simulink library "Driver_Drive_Cycle"  (R2026a)
settings: Solver=VariableStepAuto
undefined symbols (not defined in the file): Driver, Maneuver
Description:
  | Component of Simscape Vehicle Templates Library
  | 
  | Copyright 2018-2026 The MathWorks, Inc.
settings Model: Creator=smiller  LastModifiedBy=smiller

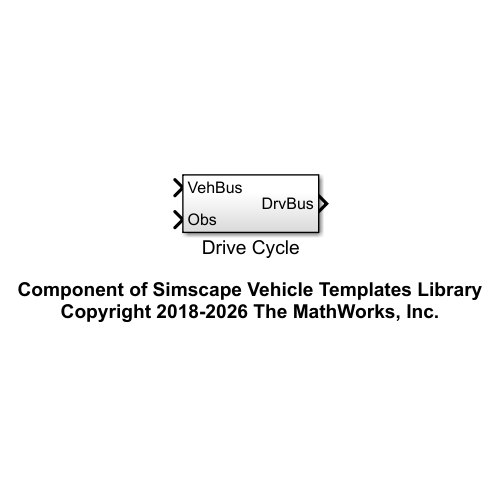
[thumbnail: Simulink's stored preview of the top-level diagram]
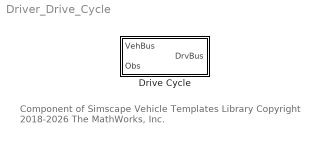
== system Driver_Drive_Cycle ==
  note: Component of Simscape Vehicle Templates Library
      | Copyright 2018-2026 The MathWorks, Inc.
  Drive Cycle : Subsystem  VariantControl=Drive_Cycle

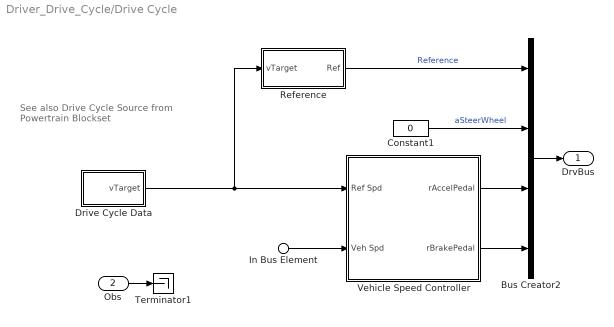
== system Driver_Drive_Cycle/Drive Cycle ==
  note: See also Drive Cycle Source
      | from Powertrain Blockset
  In Bus Element : Inport  PortName=VehBus  Element=Chassis.Body.CG.vx
  Obs : Inport  Port=2
  Bus Creator2 : BusCreator  Inputs=4
  Constant1 : Constant  Value=0
  Drive Cycle Data : Subsystem  mask{Drive_Cycle_Time=Maneuver.DriveCycle.cycle_t.Value, Drive_Cycle_Speed=Maneuver.DriveCycle.cycle_spd.Value}
      mask prompts: Drive_Cycle_Time "Drive Cycle Time (s)"; Drive_Cycle_Speed "Drive Cycle Speed (km/h)"
      mask init:
      | if(verLessThan('matlab','9.7'))
      |     set_param([gcb '/1-D Lookup Table'],'InterpMethod','Cubic spline')
      | else
      |     set_param([gcb '/1-D Lookup Table'],'InterpMethod','Akima spline')
      | end
  Reference : Subsystem
  Terminator1 : Terminator
  Vehicle Speed Controller : Subsystem  mask{Driver=Driver}
      mask prompts: Driver "Driver (structure)"
  DrvBus : Outport  VectorParamsAs1DForOutWhenUnconnected=off
  wires:
  Obs/1 -> Terminator1/1
  In Bus Element/1 -> Vehicle Speed Controller/2(Veh Spd)
  Bus Creator2/1 -> DrvBus/1
  Constant1/1 -> Bus Creator2/2  "aSteerWheel"
  Reference/1(Ref) -> Bus Creator2/1  "Reference"
  Drive Cycle Data/1(vTarget) -> Reference/1(vTarget), Vehicle Speed Controller/1(Ref Spd)
  Vehicle Speed Controller/1(rAccelPedal) -> Bus Creator2/3
  Vehicle Speed Controller/2(rBrakePedal) -> Bus Creator2/4

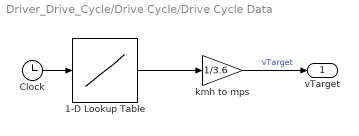
== system Driver_Drive_Cycle/Drive Cycle/Drive Cycle Data ==
  1-D Lookup Table : Lookup_n-D  NumberOfTableDimensions=1  BreakpointsForDimension1=Drive_Cycle_Time  Table=Drive_Cycle_Speed  InterpMethod=Cubic spline  InternalRulePriority=Speed  RndMeth=Simplest
  Clock : Clock
  "kmh to mps " : Gain  Gain=1/3.6
  vTarget : Outport  VectorParamsAs1DForOutWhenUnconnected=off
  wires:
  Clock/1 -> 1-D Lookup Table/1
  1-D Lookup Table/1 -> "kmh to mps "/1
  "kmh to mps "/1 -> vTarget/1  "vTarget"

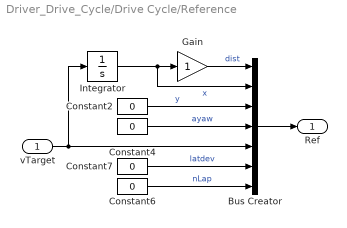
== system Driver_Drive_Cycle/Drive Cycle/Reference ==
  vTarget : Inport
  Bus Creator : BusCreator  Inputs=7
  Constant{2,4,6..7} (4 alike) : Constant  Value=0
  Gain : Gain
  Integrator : Integrator
  Ref : Outport  VectorParamsAs1DForOutWhenUnconnected=off
  wires:
  vTarget/1 -> Bus Creator/5, Integrator/1
  Constant4/1 -> Bus Creator/4  "ayaw"
  Integrator/1 -> Bus Creator/2, Gain/1  "x"
  Gain/1 -> Bus Creator/1  "dist"
  Constant2/1 -> Bus Creator/3  "y"
  Bus Creator/1 -> Ref/1
  Constant7/1 -> Bus Creator/6  "latdev"
  Constant6/1 -> Bus Creator/7  "nLap"

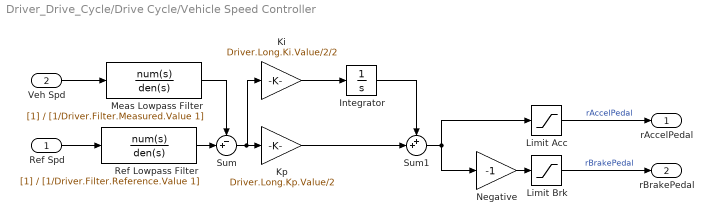
== system Driver_Drive_Cycle/Drive Cycle/Vehicle Speed Controller ==
  Ref Spd : Inport
  Veh Spd : Inport  Port=2
  Integrator : Integrator  UpperSaturationLimit=1  LowerSaturationLimit=-1  ZeroCross=off
  Ki : Gain  Gain=Driver.Long.Ki.Value/2/2
  Kp : Gain  Gain=Driver.Long.Kp.Value/2
  Limit Acc : Saturate  UpperLimit=1  LowerLimit=0  ZeroCross=off
  Limit Brk : Saturate  UpperLimit=1  LowerLimit=0  ZeroCross=off
  Meas Lowpass Filter : TransferFcn  Denominator=[1/Driver.Filter.Measured.Value 1]
  Negative : Gain  Gain=-1
  Ref Lowpass Filter : TransferFcn  Denominator=[1/Driver.Filter.Reference.Value 1]
  Sum : Sum  Inputs=-+|
  Sum1 : Sum  Inputs=++|
  rAccelPedal : Outport  VectorParamsAs1DForOutWhenUnconnected=off
  rBrakePedal : Outport  Port=2  VectorParamsAs1DForOutWhenUnconnected=off
  wires:
  Limit Acc/1 -> rAccelPedal/1  "rAccelPedal"
  Sum1/1 -> Limit Acc/1, Negative/1
  Sum/1 -> Ki/1, Kp/1
  Ki/1 -> Integrator/1
  Kp/1 -> Sum1/2
  Integrator/1 -> Sum1/1
  Veh Spd/1 -> Meas Lowpass Filter/1
  Limit Brk/1 -> rBrakePedal/1  "rBrakePedal"
  Meas Lowpass Filter/1 -> Sum/1
  Negative/1 -> Limit Brk/1
  Ref Spd/1 -> Ref Lowpass Filter/1
  Ref Lowpass Filter/1 -> Sum/2
